simulink model "12_motor_cooling_system_design_Approach2_simulink"  (R2024b)
settings: Solver=VariableStepAuto  StartTime=0.0  StopTime=240  MaxStep=0.001  RelTol=1e-3
values from neighbouring files (symbols this model uses):
  cooling = struct(     'n_tubes', 12,      'w_radiator', 0.5,      'h_tube', 0.35,      'L_tube', 0.8000,      'area_primary', 0.3000,      'area_fins', 2,      'fan_diameter', 0.4000,      'fan_thickness', 0.0500,      'cDrag', 2.5000,      'denAir', 1.2000,      'pumpArea', 0.3000,      'pipe1Length', 0.5000,      'pipe1Dia', 0.300,      'pipe2Length', 0.5000,      'pipe2Dia', 0.300  )    [MotorCoolingSystem_Parameter_Approach1.m]    (also in MotorCoolingSystem_Parameters_Approach2.m = struct(     'n_tubes', 12,      'w_radiator', 0.5,      'h_t)
libraries: fl_lib x32, nesl_utility x8, SimscapeFluids_lib x4, simulink x2
(part 1 of 3)
settings Model: Creator=JESSWIN  LastModifiedBy=JESSWIN
settings SolverCC: MaxConsecutiveMinStep=10

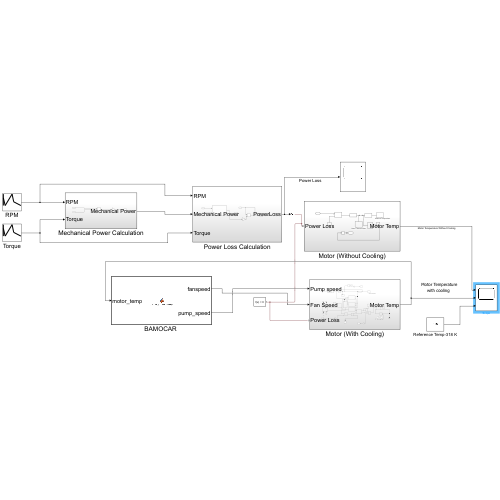
[thumbnail: Simulink's stored preview of the top-level diagram]
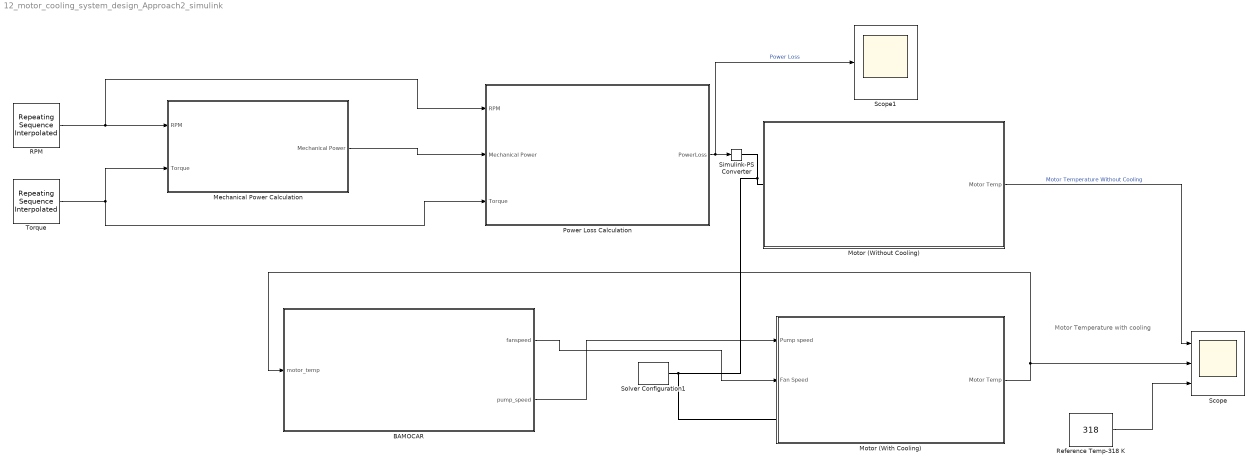
== system 12_motor_cooling_system_design_Approach2_simulink ==
  note: Motor Temperature
      | with cooling
  "BAMOCAR " : MATLAB Function  TreatAsAtomicUnit=on
  Mechanical Power Calculation : Subsystem
  Motor (With Cooling) : Subsystem
  Motor (Without Cooling) : Subsystem
  Power Loss Calculation : Subsystem
  RPM : simulink/Sources/Repeating Sequence Interpolated  OutValues=rpm  TimeValues=time  LookUpMeth=Interpolation-Use End Values  tsamp=0.01  OutMin=[]  OutMax=[]  OutDataTypeStr=double  OutputDataTypeScalingMode=double  OutDataType=fixdt(0,8)  OutScaling=2^-10
  Reference Temp-318 K : Constant  Value=318
  Scope : Scope  NumInputPorts=3
  Scope1 : Scope
  Simulink-PS Converter : nesl_utility/Simulink-PS Converter  PhysicalDomain=network_engine_domain  SubClassName=ps_input  LeftPortType=input  RightPortType=output  PseudoPeriodic=off  Frequencies=[]  NoiseDistribution=none  NoiseParameters=[]  Unit=1  AffineConversion=off  FilteringAndDerivatives=provide  SimscapeFilterOrder=1  InputFilterTimeConstant=0.001  UdotUserProvided=0
  Solver Configuration1 : nesl_utility/Solver Configuration  PhysicalDomain=network_engine_domain  SubClassName=solver  LeftPortType=input  RightPortType=generic  Tones=[]  Harmonics=[]  SimulateNoise=off  Profile=off  UseLocalSampling=off  EnableSwitchedLinearOptims=on  FrequencyDomain=off  UseCCode=off  RelTol=0.001  AbsTol=0.001  MinStep=1e-09  ToWorkspace=off  RevertToSquareIcSolve=off  NumHomotopyIterations=100  PhasorMode=off  PhasorModeNumHarmonics=1  ConsistencySolver=NEWTON_XTOL_AFTER_FTOL  IndexReductionMethod=DerivativeReplacement  DoDC=off  ResidualTolerance=1e-09  ConsistencyTolSource=GLOBAL  ConsistencyAbsTol=0.001  ConsistencyRelTol=0.001  ConsistencyTolFactor=0.001  UseLocalSolver=off  LocalSolverChoice=NE_BACKWARD_EULER_ADVANCER  ResolveIndetEquations=on  FunctionEvalNumThread=1  LocalSolverSampleTime=0.001  DoFixedCost=off  MaxNonlinIter=3  MaxModeIter=2  ComputeImpulses=off  ImpulseIterations=2  LinearAlgebra=auto  LinearAlgebraNumThread=0  EquationFormulation=NE_TIME_EF  DelaysMemoryBudget=1024  AutomaticFiltering=on  FilteringTimeConstant=0.001  PartitionStorageMethod=AS_NEEDED  PartitionMemoryBudget=1024  PartitionMethod=ROBUST  MultibodyUseLocalSolver=off  MultibodyLocalSolverChoice=ODE1  MultibodyLocalSolverSampleTime=0.001
  Torque : simulink/Sources/Repeating Sequence Interpolated  OutValues=torque  TimeValues=time  LookUpMeth=Interpolation-Use End Values  tsamp=0.01  OutMin=[]  OutMax=[]  OutDataTypeStr=double  OutputDataTypeScalingMode=double  OutDataType=fixdt(0,8)  OutScaling=2^-10
  wires:
  RPM/1 -> Power Loss Calculation/1(RPM), Mechanical Power Calculation/1(RPM)
  Torque/1 -> Power Loss Calculation/3(Torque), Mechanical Power Calculation/2(Torque)
  Motor (With Cooling)/1(Motor Temp) -> "BAMOCAR "/1(motor_temp), Scope/2
  "BAMOCAR "/2(pump_speed) -> Motor (With Cooling)/1(Pump speed)
  Reference Temp-318 K/1 -> Scope/3
  Mechanical Power Calculation/1(Mechanical Power) -> Power Loss Calculation/2(Mechanical Power)
  Power Loss Calculation/1(PowerLoss) -> Scope1/1, Simulink-PS Converter/1  "Power Loss"
  "BAMOCAR "/1(fanspeed) -> Motor (With Cooling)/2(Fan Speed)
  Motor (Without Cooling)/1(Motor Temp) -> Scope/1  "Motor Temperature Without Cooling"
  connections:
  Simulink-PS Converter/RConn1 -- Solver Configuration1/RConn1 -- Motor (With Cooling)/LConn1 -- Motor (Without Cooling)/LConn1

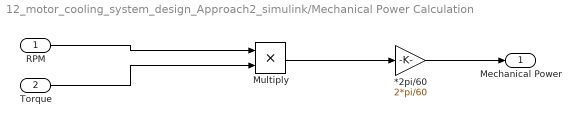
== system 12_motor_cooling_system_design_Approach2_simulink/Mechanical Power Calculation ==
  RPM : Inport
  Torque : Inport  Port=2
  *2pi/60 : Gain  Gain=2*pi/60
  Multiply : Product
  Mechanical Power : Outport
  wires:
  Multiply/1 -> *2pi/60/1
  *2pi/60/1 -> Mechanical Power/1
  RPM/1 -> Multiply/1
  Torque/1 -> Multiply/2
